simulink model "Simscape_motor_propeller_model"  (R2019b)
settings: Solver=FixedStepDiscrete  StartTime=0.0  StopTime=5  RelTol=1e-3
undefined symbols (not defined in the file or in its folder): DiscIntNeverNeededParam
libraries: fl_lib x6, nesl_utility x5, ee_lib x1
settings Model: Creator=Anas  LastModifiedBy=Anas
settings SolverCC: ZeroCrossAlgorithm=Adaptive
settings OptimizationCC: BlockReduction=off  ConditionallyExecuteInputs=off  DefaultParameterBehavior=Inlined
settings DebuggingCC: AlgebraicLoopMsg=error  IgnoredZcDiagnostic=none  SingleTaskRateTransMsg=error
settings HardwareCC: ProdBitPerPointer=32  ProdBitPerSizeT=32  ProdBitPerPtrDiffT=32  ProdLargestAtomicFloat=None  ProdIntDivRoundTo=Undefined  ProdEndianess=Unspecified  ProdWordSize=32  ProdHWDeviceType=ASIC/FPGA->ASIC/FPGA  TargetBitPerPointer=64  TargetBitPerSizeT=64  TargetBitPerPtrDiffT=64  TargetLongLongMode=on  TargetIntDivRoundTo=Zero  TargetEndianess=LittleEndian  TargetWordSize=64  TargetHWDeviceType=Custom Processor->MATLAB Host Computer  ProdEqTarget=off

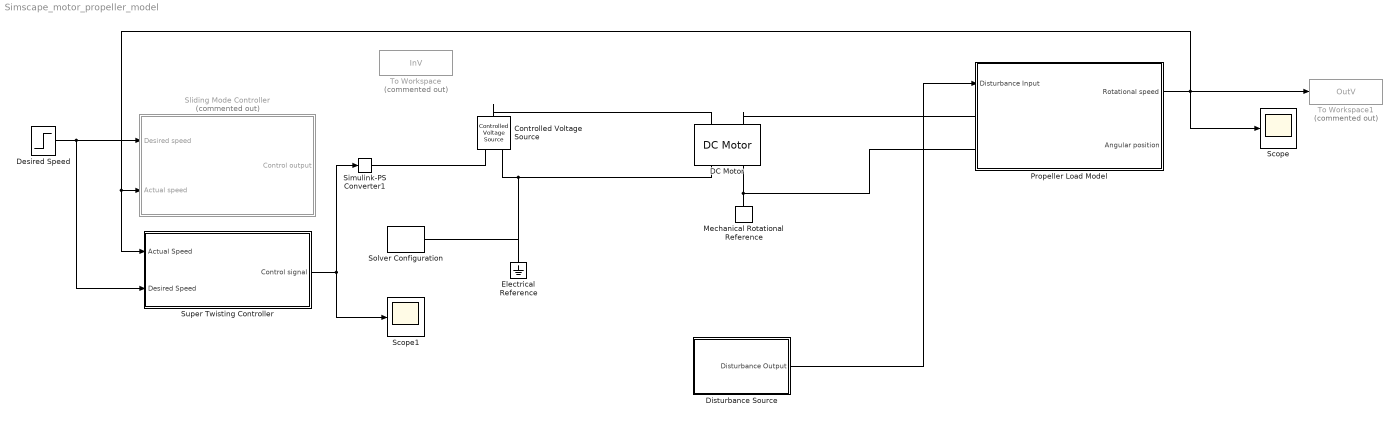
== system Simscape_motor_propeller_model ==
  Controlled Voltage Source : fl_lib/Electrical/Electrical Sources/Controlled Voltage Source
  DC Motor : ee_lib/Electromechanical/Brushed Motors/DC Motor  parameterization=3  Ra=3.9 Ohm  La=12e-6 H  emf_or_torque=1  Kv=0.072e-3 V/rpm  Ki=6.876e-4 N*m/A  T_stall=0.24e-3 N*m  w_max=9100 rpm  w_rated=4500 rpm  P_rated=0.462 W  V_rated=6.0 V  J=1e-9 g*cm^2  lam_param=2  lam=0 N*m/(rad/s)  i_noload=70 mA  V_i_noload=6.0 V  speed0=0 rpm  alpha=3.93e-3 1/K  Tmeas=25 degC  thermal_mass=100 J/K  initial_temperature=25 degC
      settings: SourceProductName=Simscape Electrical  LogSimulationData=on
  Desired Speed : Step  Time=0  After=600  SampleTime=0
  Disturbance Source : Subsystem  VariantControl=Variant1  mask{StepTime=0.2, Tmax=0.0001, Bias=0, Freq=314}
      mask prompts: StepTime "Step Time (s)"; Tmax "Torque (N.m)"; Bias "Bias (N.m)"; Freq "Frequency (rad/s)"
  Electrical Reference : fl_lib/Electrical/Electrical Elements/Electrical Reference
  Mechanical Rotational Reference : fl_lib/Mechanical/Rotational Elements/Mechanical Rotational Reference
  Propeller Load Model : Subsystem  mask{T=0.00098, J=5e-8, e=0}
      mask prompts: T "Torque (N.m)"; J "Inertia (Kg.m^2)"; e "Coupling Delay"
  Scope : Scope
  Scope1 : Scope
  Simulink-PS Converter1 : nesl_utility/Simulink-PS Converter  PhysicalDomain=network_engine_domain  SubClassName=ps_input  LeftPortType=input  RightPortType=output  PseudoPeriodic=off  Frequencies=[]  NoiseDistribution=none  NoiseParameters=[]  Unit=1  AffineConversion=off  FilteringAndDerivatives=provide  SimscapeFilterOrder=1  InputFilterTimeConstant=0.001  UdotUserProvided=0
  Sliding Mode Controller : Subsystem  Commented=on
  Solver Configuration : nesl_utility/Solver Configuration  PhysicalDomain=network_engine_domain  SubClassName=solver  LeftPortType=input  RightPortType=generic  Tones=[]  Harmonics=[]  SimulateNoise=off  Profile=off  UseLocalSampling=off  EnableSwitchedLinearOptims=on  FrequencyDomain=off  UseCCode=off  RelTol=0.001  AbsTol=1e-06  MinStep=1e-09  ToWorkspace=off  RevertToSquareIcSolve=off  NumHomotopyIterations=100  PhasorMode=off  PhasorModeNumHarmonics=1  DoDC=off  ResidualTolerance=1e-09  UseLocalSolver=off  LocalSolverChoice=NE_BACKWARD_EULER_ADVANCER  LocalSolverSampleTime=0.001  DoFixedCost=off  MaxNonlinIter=3  MaxModeIter=2  LinearAlgebra=auto  EquationFormulation=NE_TIME_EF  DelaysMemoryBudget=1024  AutomaticFiltering=on  FilteringTimeConstant=0.001  PartitionStorageMethod=AS_NEEDED  PartitionMemoryBudget=1024  PartitionMethod=ROBUST
  Super Twisting Controller : Subsystem
  To Workspace : ToWorkspace  Commented=on  VariableName=InV  SaveFormat=Timeseries  SampleTime=-1
      settings: Save2DSignal=2-D array (concatenate along first dimension)
  To Workspace1 : ToWorkspace  Commented=on  VariableName=OutV  SaveFormat=Timeseries  SampleTime=-1
  wires:
  Disturbance Source/1("Disturbance Output ") -> Propeller Load Model/1(Disturbance Input)
  Propeller Load Model/1(Rotational speed) -> To Workspace1/1, Super Twisting Controller/1(Actual Speed), Sliding Mode Controller/2(Actual speed), Scope/1
  Desired Speed/1 -> Super Twisting Controller/2(Desired Speed), Sliding Mode Controller/1(Desired speed)
  Super Twisting Controller/1(Control signal) -> Scope1/1, Simulink-PS Converter1/1
  connections:
  Solver Configuration/RConn1 -- Electrical Reference/LConn1 -- Controlled Voltage Source/RConn2 -- DC Motor/RConn1
  Mechanical Rotational Reference/LConn1 -- Propeller Load Model/LConn2 -- DC Motor/RConn2
  Controlled Voltage Source/LConn1 -- DC Motor/LConn1
  Simulink-PS Converter1/RConn1 -- Controlled Voltage Source/RConn1
  DC Motor/LConn2 -- Propeller Load Model/LConn1

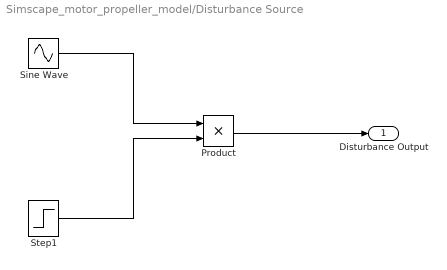
== system Simscape_motor_propeller_model/Disturbance Source ==
  Product : Product
  Sine Wave : Sin  Amplitude=Tmax  Bias=Bias  Frequency=Freq  SampleTime=0
  Step1 : Step  Time=StepTime  SampleTime=0
  "Disturbance Output " : Outport
  wires:
  Sine Wave/1 -> Product/1
  Step1/1 -> Product/2
  Product/1 -> "Disturbance Output "/1

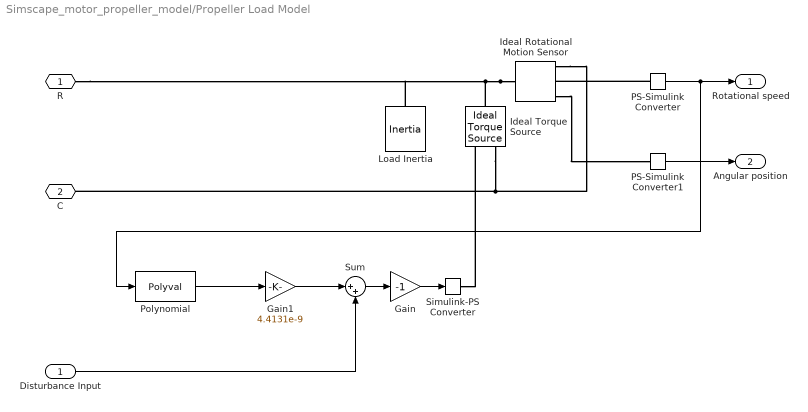
== system Simscape_motor_propeller_model/Propeller Load Model ==
  Disturbance Input : Inport
  Gain : Gain  Gain=-1
  Gain1 : Gain  Gain=4.4131e-9
  Ideal Rotational Motion Sensor : fl_lib/Mechanical/Mechanical Sensors/Ideal Rotational Motion Sensor  offset=0 rad
  Ideal Torque Source : fl_lib/Mechanical/Mechanical Sources/Ideal Torque Source
  Load Inertia : fl_lib/Mechanical/Rotational Elements/Inertia  inertia=J kg*m^2  w_specify=off  w_priority=High  w=0 rad/s  w_nominal_specify=off  w_nominal_unit=rad/s  w_nominal_value=1  t_specify=off  t_priority=None  t=0 N*m  t_nominal_specify=off  t_nominal_unit=N*m  t_nominal_value=1
  PS-Simulink Converter : nesl_utility/PS-Simulink Converter  PhysicalDomain=network_engine_domain  SubClassName=ps_output  LeftPortType=input  RightPortType=output  PseudoPeriodic=off  Frequencies=[]  Unit=inherit  AffineConversion=off
  PS-Simulink Converter1 : nesl_utility/PS-Simulink Converter  PhysicalDomain=network_engine_domain  SubClassName=ps_output  LeftPortType=input  RightPortType=output  PseudoPeriodic=off  Frequencies=[]  Unit=inherit  AffineConversion=off
  Polynomial : Polyval  Coefs=[1 0 0 ]
  Simulink-PS Converter : nesl_utility/Simulink-PS Converter  PhysicalDomain=network_engine_domain  SubClassName=ps_input  LeftPortType=input  RightPortType=output  PseudoPeriodic=off  Frequencies=[]  NoiseDistribution=none  NoiseParameters=[]  Unit=1  AffineConversion=off  FilteringAndDerivatives=provide  SimscapeFilterOrder=1  InputFilterTimeConstant=0.001  UdotUserProvided=0
  Sum : Sum  Inputs=|++
  R : PMIOPort  Side=Left
  C : PMIOPort  Port=2  Side=Left
  Rotational speed : Outport
  Angular position : Outport  Port=2
  wires:
  Disturbance Input/1 -> Sum/2
  Gain/1 -> Simulink-PS Converter/1
  Sum/1 -> Gain/1
  Gain1/1 -> Sum/1
  PS-Simulink Converter/1 -> Polynomial/1, Rotational speed/1
  PS-Simulink Converter1/1 -> Angular position/1
  Polynomial/1 -> Gain1/1
  connections:
  Ideal Rotational Motion Sensor/LConn1 -- R/RConn1 -- Load Inertia/LConn1 -- Ideal Torque Source/LConn1
  Ideal Rotational Motion Sensor/RConn1 -- C/RConn1 -- Ideal Torque Source/RConn2
  Simulink-PS Converter/RConn1 -- Ideal Torque Source/RConn1
  PS-Simulink Converter/LConn1 -- Ideal Rotational Motion Sensor/RConn2
  Ideal Rotational Motion Sensor/RConn3 -- PS-Simulink Converter1/LConn1

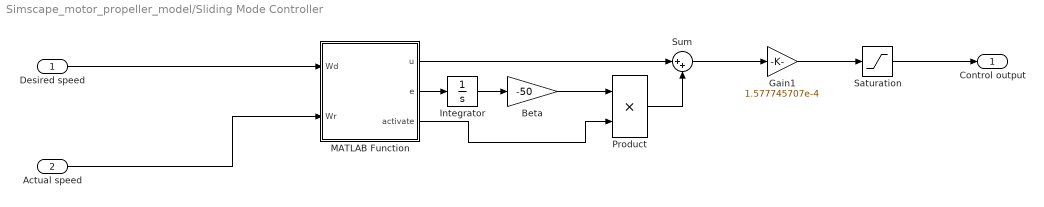
== system Simscape_motor_propeller_model/Sliding Mode Controller ==
  Desired speed : Inport
  Actual speed : Inport  Port=2
  Beta : Gain  Gain=-50
  Gain1 : Gain  Gain=1.577745707e-4
  Integrator : Integrator
  MATLAB Function : MATLAB Function  TreatAsAtomicUnit=on
  Product : Product
  Saturation : Saturate  UpperLimit=11  LowerLimit=-11
  Sum : Sum  Inputs=|++
  Control output : Outport
  wires:
  Actual speed/1 -> MATLAB Function/2(Wr)
  Gain1/1 -> Saturation/1
  Desired speed/1 -> MATLAB Function/1(Wd)
  Saturation/1 -> Control output/1
  MATLAB Function/2(e) -> Integrator/1
  Integrator/1 -> Beta/1
  Sum/1 -> Gain1/1
  MATLAB Function/1(u) -> Sum/1
  MATLAB Function/3(activate) -> Product/2
  Beta/1 -> Product/1
  Product/1 -> Sum/2

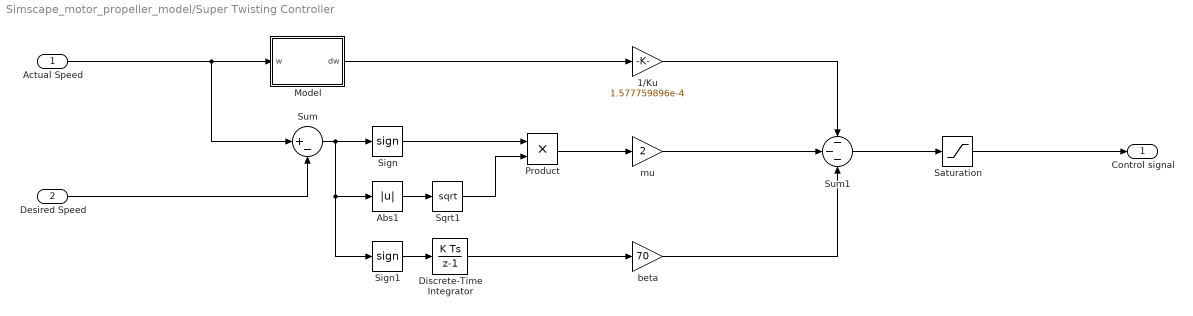
== system Simscape_motor_propeller_model/Super Twisting Controller ==
  Actual Speed : Inport  Unit=rad/sec
  Desired Speed : Inport  Port=2
  1/Ku : Gain  Gain=1.577759896e-4
  Abs1 : Abs
  Discrete-Time Integrator : DiscreteIntegrator  SampleTime=-1  OutDataTypeStr=double  ICPrevOutput=DiscIntNeverNeededParam  ICPrevScaledInput=DiscIntNeverNeededParam
  Model : MATLAB Function  TreatAsAtomicUnit=on
  Product : Product
  Saturation : Saturate  UpperLimit=11  LowerLimit=-11
  Sign : Signum
  Sign1 : Signum
  Sqrt1 : Sqrt  IntermediateResultsDataTypeStr=double  SaturateOnIntegerOverflow=on
  Sum : Sum  Inputs=|+-
  Sum1 : Sum  Inputs=---
  beta : Gain  Gain=70
  mu : Gain  Gain=2
  Control signal : Outport  VectorParamsAs1DForOutWhenUnconnected=off
  wires:
  Sum1/1 -> Saturation/1
  Product/1 -> mu/1
  mu/1 -> Sum1/2
  Actual Speed/1 -> Sum/1, Model/1(w)
  Discrete-Time Integrator/1 -> beta/1
  beta/1 -> Sum1/3
  Sign1/1 -> Discrete-Time Integrator/1
  Model/1(dw) -> 1/Ku/1
  Sum/1 -> Abs1/1, Sign1/1, Sign/1
  Sign/1 -> Product/1
  Desired Speed/1 -> Sum/2
  Abs1/1 -> Sqrt1/1
  Sqrt1/1 -> Product/2
  Saturation/1 -> Control signal/1
  1/Ku/1 -> Sum1/1

== matlab function Simscape_motor_propeller_model/Super Twisting Controller/Model ==
  data: w input; dw output
function dw = Model(w)
%System Model
dw=-0.08653*w^2-39.902*w;
end

== matlab function Simscape_motor_propeller_model/Sliding Mode Controller/MATLAB Function ==
  data: Wd input; u output; Wr input; e output; activate output
function [u,e,activate] = SMC(Wd,Wr)
%Sliding mode controller for a motor-propeller system
%Model
function y=f(x)
        y=-0.08653*x^2-39.902*x;
end
e=Wr-Wd;
mu=20;
Ku=6338.1;
static=Ku*8.6921948;
activate=1;
u=(-f(Wr)-Ku*mu*sign(e)*sqrt(abs(e)))*activate+static*(1-activate);
end
